simulink model "SiDrivetrain"  (R2020a)
settings: Solver=ode23tb  StartTime=0.0  StopTime=50  RelTol=1e-3  EnableMultiTasking=on
model workspace (MAT data in the model file):
  N = [-4.7 4.75 4.75 3.75 3.25 2.75 2.25 1.5 1 0.75]
  NF = Simulink.Parameter
  NF.Value = 2
  NF.DataType = 'auto'
  NF.Dimensions = [1 1]
  NR = Simulink.Parameter
  NR.Value = 2
  NR.DataType = 'auto'
  NR.Dimensions = [1 1]
  Ndiff = 3
  RWheel = 0.3
  b_axle = Simulink.Parameter
  b_axle.Value = 10
  b_axle.DataType = 'auto'
  b_axle.Dimensions = [1 1]
  b_driveshaft = Simulink.Parameter
  b_driveshaft.Value = 10
  b_driveshaft.DataType = 'auto'
  b_driveshaft.Dimensions = [1 1]
  dt_DCT = Simulink.Parameter
  dt_DCT.Value = 0.001
  dt_DCT.DataType = 'auto'
  dt_DCT.Dimensions = [1 1]
  k_axle = Simulink.Parameter
  k_axle.Value = 5000
  k_axle.DataType = 'auto'
  k_axle.Dimensions = [1 1]
  k_driveshaft = Simulink.Parameter
  k_driveshaft.Value = 1000
  k_driveshaft.DataType = 'auto'
  k_driveshaft.Dimensions = [1 1]
  k_hyd = Simulink.Parameter
  k_hyd.Value = 5000000
  k_hyd.DataType = 'auto'
  k_hyd.Dimensions = [1 1]
  tau_hyd = Simulink.Parameter
  tau_hyd.Value = 0.01
  tau_hyd.DataType = 'auto'
  tau_hyd.Dimensions = [1 1]
  wc_shaft = Simulink.Parameter
  wc_shaft.Value = 300
  wc_shaft.DataType = 'auto'
  wc_shaft.Dimensions = [1 1]
values from neighbouring files (symbols this model uses):
  b_axle = 10.0    [DrivetrainEvDD.sldd]    (also in DrivetrainHevMmDD.sldd; SiDrivetrainDD.sldd)
  b_driveshaft = 10.0    [DrivetrainEvDD.sldd]    (also in DrivetrainHevMmDD.sldd; SiDrivetrainDD.sldd)
  k_axle = 5000.0    [DrivetrainEvDD.sldd]    (also in DrivetrainHevMmDD.sldd; SiDrivetrainDD.sldd)
  k_driveshaft = 1000.0    [DrivetrainEvDD.sldd]    (also in DrivetrainHevMmDD.sldd; SiDrivetrainDD.sldd)
libraries: autolibsharedcoupling x12, autolibpowerinfoutils x6, autolibshareddiff x4, autolibutils x3, autolibshared x3, autolibcoupling x2, simulink x2, autolibsharedtransfixedgear x2, autolibtransdct x1, autolibshareddrivetraincommon x1, autolibtranscontrols x1
(part 1 of 4)
settings Model: ModifiedByFormat=The MathWorks, Inc.  PauseTimes=9  Creator=The MathWorks, Inc.  LastModifiedBy=The MathWorks, Inc.
settings SolverCC: DecoupledContinuousIntegration=on
settings DataIOCC: DSMLogging=off  ReturnWorkspaceOutputs=off
settings DebuggingCC: MergeDetectMultiDrivingBlocksExec=none  ArithmeticOperatorsInVariantConditions=warning
settings ModelReferenceCC: PropagateSignalLabelsOutOfModel=off
settings SFSimCC: SimUseLocalCustomCode=off
settings RTWCC: RTWUseLocalCustomCode=off
settings CodeAppCC: StateflowObjectComments=on
settings GRTTargetCC: TargetLangStandard=C89/C90 (ANSI)
settings ConfigComp: CovMetricSettings=dsw  CovHtmlReporting=on  CovSaveCumulativeToWorkspaceVar=on  CovSaveSingleToWorkspaceVar=on  CovShowResultsExplorer=off  CovExternalEMLEnable=off
settings SimscapeCC: SimscapeNormalizeSystem=off  SimscapeNominalValues={1, 'bar'; 1, 'cm^3/s'; 1, 'bar*kg/s'; 1, 'kJ/kg'; 1, 'kW'; }

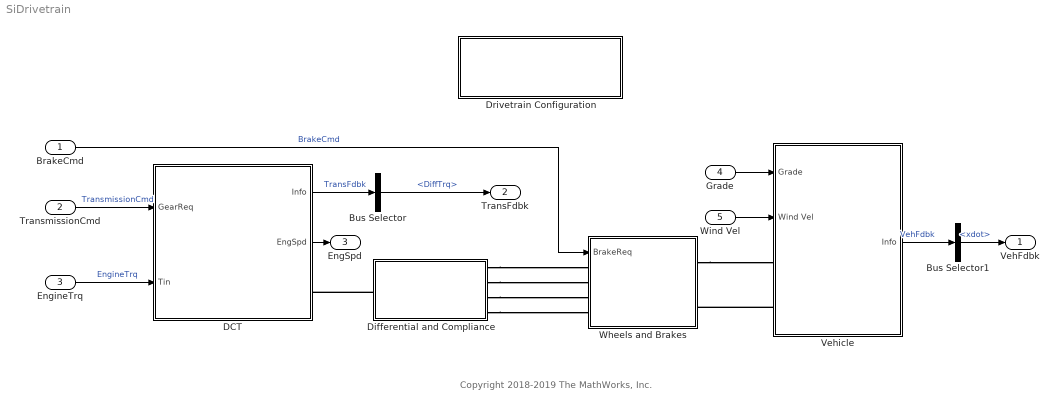
== system SiDrivetrain ==
  note: Copyright 2018-2019 The MathWorks, Inc.
  BrakeCmd : Inport
  TransmissionCmd : Inport  Port=2
  EngineTrq : Inport  Port=3
  Grade : Inport  Port=4
  Wind Vel : Inport  Port=5
  Bus Selector : BusSelector  OutputSignals=Diff.DiffTrq
  Bus Selector1 : BusSelector  OutputSignals=BdyFrm.Cg.Vel.xdot
  DCT : Subsystem  Variant=on  VariantControlMode=Label  LabelModeActiveChoice=0
  Differential and Compliance : Subsystem  Variant=on  VariantControlMode=Label  LabelModeActiveChoice=0
  Drivetrain Configuration : Subsystem  mask(Drivetrain Configuration){drivetrainMode=Front Wheel Drive}
      mask prompts: drivetrainMode "Drivetrain Mode"
      mask help: Use this block to configure the dirvetrain mode.
      settings: AttributesFormatString=Active Mode: %<drivetrainMode>
      mask TypeOptions drivetrainMode: Front Wheel Drive | Rear Wheel Drive | All Wheel Drive
      mask Callback drivetrainMode:
      | switch get_param(gcb,'drivetrainMode')
      |     case 'Front Wheel Drive'
      |         set_param([bdroot '/Differential and Compliance'],'OverrideUsingVariant','0')
      |     case 'Rear Wheel Drive'
      |         set_param([bdroot '/Differential and Compliance'],'OverrideUsingVariant','1')
      |     case 'All Wheel Drive'
      |         set_param([bdroot '/Differential and Compliance'],'OverrideUsingVariant','2')
      |     otherwise
      |         set_param([bdroot '/Differential and Compliance'],'OverrideUsingVariant','0')
      | end
      mask Display: disp('Double click to configure drivetrain')
  Vehicle : Subsystem
  Wheels and Brakes : Subsystem  VariantControl=0
  VehFdbk : Outport  VectorParamsAs1DForOutWhenUnconnected=off
  TransFdbk : Outport  Port=2  VectorParamsAs1DForOutWhenUnconnected=off  BusOutputAsStruct=on
  EngSpd : Outport  Port=3  VectorParamsAs1DForOutWhenUnconnected=off  BusOutputAsStruct=on
  wires:
  Vehicle/1(Info) -> Bus Selector1/1  "VehFdbk"
  BrakeCmd/1 -> Wheels and Brakes/1(BrakeReq)  "BrakeCmd"
  Bus Selector1/1 -> VehFdbk/1  "<xdot>"
  Bus Selector/1 -> TransFdbk/1  "<DiffTrq>"
  TransmissionCmd/1 -> DCT/1(GearReq)  "TransmissionCmd"
  DCT/1(Info) -> Bus Selector/1  "TransFdbk"
  DCT/2(EngSpd) -> EngSpd/1
  EngineTrq/1 -> DCT/2(Tin)  "EngineTrq"
  Grade/1 -> Vehicle/1(Grade)
  Wind Vel/1 -> Vehicle/2(Wind Vel)
  connections:
  Differential and Compliance/LConn1 -- DCT/RConn1
  Differential and Compliance/RConn4 -- Wheels and Brakes/LConn4
  Vehicle/LConn2 -- Wheels and Brakes/RConn2
  Differential and Compliance/RConn3 -- Wheels and Brakes/LConn3
  Differential and Compliance/RConn2 -- Wheels and Brakes/LConn2
  Differential and Compliance/RConn1 -- Wheels and Brakes/LConn1
  Wheels and Brakes/RConn1 -- Vehicle/LConn1

== system SiDrivetrain/DCT ==
  note: 1) Add Subsystem or Model blocks as valid variant choices.
      | 2) You cannot connect blocks at this level. At simulation, connectivity is automatically
      | determined, based on the active variant and port name matching.
  GearReq : Inport
  Tin : Inport  Port=2
  DCT Block : Subsystem  VariantControl=0
      settings: MinAlgLoopOccurrences=on
  DCT System : Subsystem  VariantControl=1
      settings: MinAlgLoopOccurrences=on
  T : PMIOPort  Side=Right
  Info : Outport  VectorParamsAs1DForOutWhenUnconnected=off
  EngSpd : Outport  Port=2  VectorParamsAs1DForOutWhenUnconnected=off

== system SiDrivetrain/Differential and Compliance ==
  All Wheel Drive : Subsystem  VariantControl=2
  Front Wheel Drive : Subsystem  VariantControl=0
  Rear Wheel Drive : Subsystem  VariantControl=1
  D : PMIOPort  Side=Left
  FA1 : PMIOPort  Port=2  Side=Right
  FA2 : PMIOPort  Port=3  Side=Right
  RA1 : PMIOPort  Port=4  Side=Right
  RA2 : PMIOPort  Port=5  Side=Right

== system SiDrivetrain/Drivetrain Configuration ==

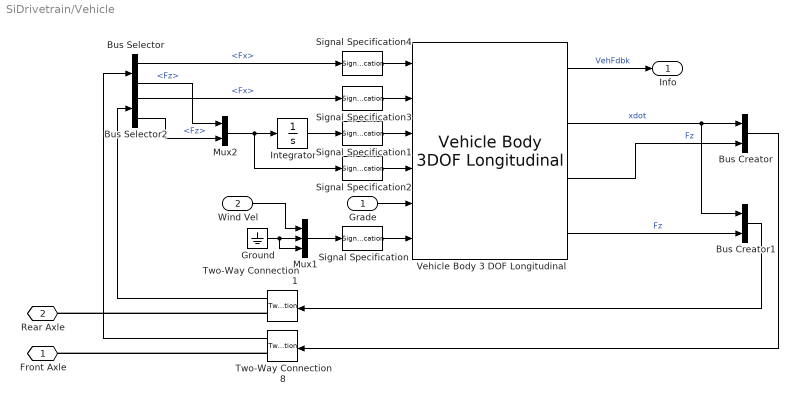
== system SiDrivetrain/Vehicle ==
  Grade : Inport  Unit=deg
  Wind Vel : Inport  Port=2  Unit=m/s
  Bus Creator : BusCreator  Inputs=2
  Bus Creator1 : BusCreator  Inputs=2
  Bus Selector : BusSelector  OutputSignals=Fx,Fz
  Bus Selector2 : BusSelector  OutputSignals=Fx,Fz
  Ground : Ground
  Integrator : Integrator
  Mux1 : Mux  Inputs=3
  Mux2 : Mux  Inputs=2
  Signal Specification : SignalSpecification  Unit=m/s
  Signal Specification1 : SignalSpecification  Unit=m
  Signal Specification2 : SignalSpecification  Unit=m/s
  Signal Specification3 : SignalSpecification  Unit=N
  Signal Specification4 : SignalSpecification  Unit=N
  Two-Way Connection1 : TwoWayConnection
  Two-Way Connection8 : TwoWayConnection
  Vehicle Body 3 DOF Longitudinal : autolibshared/Vehicle Body 3DOF Longitudinal  VariantControl=SL  groundType=Axle displacement, velocity  aMode=1  extFMode=off  extMMode=off  extTamb=off  NF=NF  NR=NR  m=1200  a=1.4  b=1.8  h=.35  Cd=.3  Af=2  x_o=0  xdot_o=0  Cl=.1  z_o=-.35  zdot_o=0  Iyy=3000  Cpm=.1  theta_o=0  q_o=0  FskF=[-50, -1, 0, 2, 3, 52].*1.25e4  dzsF=[-5e-3, -1e-4, 0, .2, .2001, .2051]  FsbF=[-10000 -100 -10 0 10 100 10000]  dzdotsF=[-10 -1 -.1 0 .1 1 10]  FskR=[-50, -1, 0, 2, 3, 52].*7.5e3  dzsR=[-5e-3, -1e-4, 0, .2, .2001, .2051]  FsbR=[-10000 -100 -10 0 10 100 10000]  dzdotsR=[-10 -1 -.1 0 .1 1 10]  Pabs=101325  T=273  g=9.81  blkID=0
      settings: SourceProductBaseCode=PW,MT,VE,VP
  Front Axle : PMIOPort  Side=Left
  Rear Axle : PMIOPort  Port=2  Side=Left
  Info : Outport  VectorParamsAs1DForOutWhenUnconnected=off
  wires:
  Vehicle Body 3 DOF Longitudinal/3 -> Bus Creator/2  "Fz"
  Vehicle Body 3 DOF Longitudinal/2 -> Bus Creator1/1, Bus Creator/1  "xdot"
  Two-Way Connection8/1 -> Bus Selector/1
  Vehicle Body 3 DOF Longitudinal/1 -> Info/1  "VehFdbk"
  Ground/1 -> Mux1/2, Mux1/3
  Mux1/1 -> Signal Specification/1
  Vehicle Body 3 DOF Longitudinal/4 -> Bus Creator1/2  "Fz"
  Mux2/1 -> Integrator/1, Signal Specification2/1
  Integrator/1 -> Signal Specification1/1
  Wind Vel/1 -> Mux1/1
  Grade/1 -> Vehicle Body 3 DOF Longitudinal/5
  Signal Specification/1 -> Vehicle Body 3 DOF Longitudinal/6
  Signal Specification1/1 -> Vehicle Body 3 DOF Longitudinal/3
  Signal Specification2/1 -> Vehicle Body 3 DOF Longitudinal/4
  Signal Specification3/1 -> Vehicle Body 3 DOF Longitudinal/2
  Signal Specification4/1 -> Vehicle Body 3 DOF Longitudinal/1
  Bus Creator/1 -> Two-Way Connection8/1
  Bus Creator1/1 -> Two-Way Connection1/1
  Bus Selector/1 -> Signal Specification4/1  "<Fx>"
  Bus Selector/2 -> Mux2/1  "<Fz>"
  Bus Selector2/1 -> Signal Specification3/1  "<Fx>"
  Bus Selector2/2 -> Mux2/2  "<Fz>"
  Two-Way Connection1/1 -> Bus Selector2/1
  connections:
  Two-Way Connection8/RConn1 -- Front Axle/RConn1
  Two-Way Connection1/RConn1 -- Rear Axle/RConn1
